simulink model "lab1_s"  (R2022b)
settings: Solver=VariableStepAuto  StartTime=0.0  StopTime=30  RelTol=1e-3
libraries: dspsrcs4 x2
settings Model: Creator=Est01  LastModifiedBy=MIGUEL

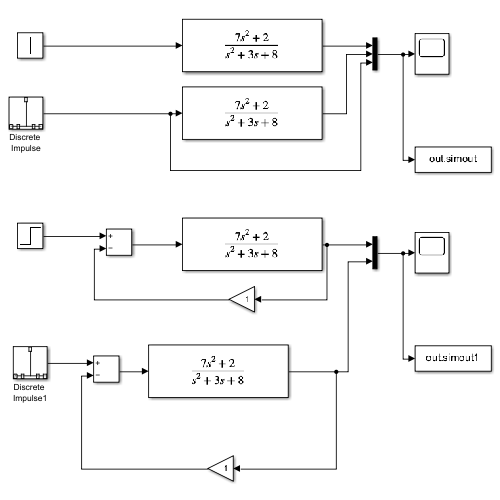
[thumbnail: Simulink's stored preview of the top-level diagram]
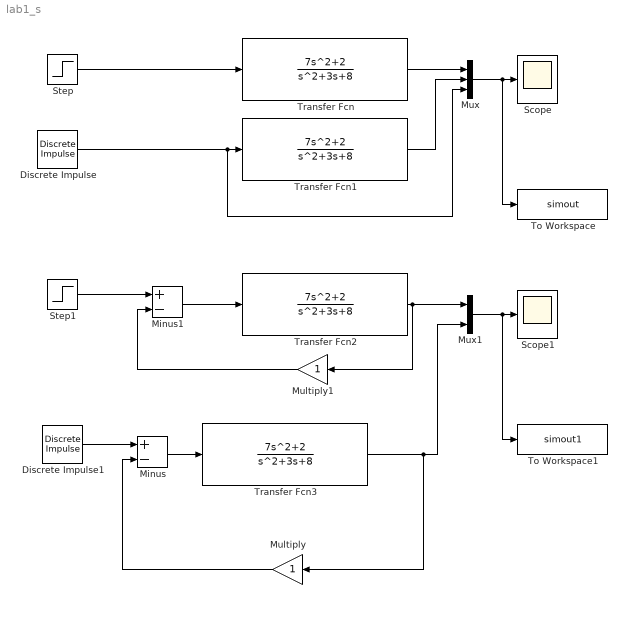
== system lab1_s ==
  Discrete Impulse : dspsrcs4/Discrete  Impulse  Delay=0  SampleTime=0.1  FrameSample=1  OutputFrames=off  dataType=double  isSigned=on  wordLen=16  udDataType=sfix(16)  fracBitsMode=Best precision  numFracBits=15  OutDataTypeStr=double  LastOutDataTypeStr=double
  Discrete Impulse1 : dspsrcs4/Discrete  Impulse  Delay=0  SampleTime=0.1  FrameSample=1  OutputFrames=off  dataType=double  isSigned=on  wordLen=16  udDataType=sfix(16)  fracBitsMode=Best precision  numFracBits=15  OutDataTypeStr=double  LastOutDataTypeStr=double
  Minus : Sum  Inputs=+-
  Minus1 : Sum  Inputs=+-
  Multiply : Gain
  Multiply1 : Gain
  Mux : Mux  Inputs=3
  Mux1 : Mux  Inputs=2
  Scope : Scope
  Scope1 : Scope
  Step : Step  Time=0  SampleTime=0
  Step1 : Step  Time=0  SampleTime=0
  To Workspace : ToWorkspace  VariableName=simout  SaveFormat=Structure With Time  SampleTime=-1
  To Workspace1 : ToWorkspace  VariableName=simout1  SaveFormat=Structure With Time  SampleTime=-1
  Transfer Fcn{,1..3} (4 alike) : TransferFcn  Numerator=[7 0 2]  Denominator=[1 3 8]
  wires:
  Transfer Fcn/1 -> Mux/1
  Mux/1 -> To Workspace/1, Scope/1
  Step/1 -> Transfer Fcn/1
  Discrete Impulse/1 -> Mux/3, Transfer Fcn1/1
  Transfer Fcn1/1 -> Mux/2
  Mux1/1 -> To Workspace1/1, Scope1/1
  Transfer Fcn3/1 -> Multiply/1, Mux1/2
  Transfer Fcn2/1 -> Multiply1/1, Mux1/1
  Multiply/1 -> Minus/2
  Discrete Impulse1/1 -> Minus/1
  Minus/1 -> Transfer Fcn3/1
  Multiply1/1 -> Minus1/2
  Step1/1 -> Minus1/1
  Minus1/1 -> Transfer Fcn2/1
